simulink model "slosh_control_loop"  (R2025b)
settings: Solver=ode45  StartTime=0.0  StopTime=20  RelTol=1e-3
values from neighbouring files (symbols this model uses):
  A_mimo = A    [LQR_Tuning.m]
  A_slosh = [0, 1; -k_slosh/m_slosh_comp, -b_slosh/m_slosh_comp]    [adaptive_pid_vs_lqi_comparison.m]    (also in comprehensive_slosh_analysis.m = [0, 1; -k_slosh_comp/m_slosh_comp, -b_slosh_comp/m_slosh_com; improved_physics_slosh_model.m; separated_architecture.m = [0,                1; separated_system_params.mat = [0  1; -4  -0.2])
  B_nom = [B_mimo,B_nom(:,3),B_nom(:,4)]    [LQR_Tuning.m]    (also in adaptive_pid_vs_lqi_comparison.m = [0,     0; comprehensive_slosh_analysis.m = [0,     0; improved_physics_slosh_model.m = [0,     0; separated_architecture.m = [1/m_aircraft,  XT/m_aircraft, 1/m_aircraft,      0)
  B_slosh = [0; 1]    [adaptive_pid_vs_lqi_comparison.m]    (also in comprehensive_slosh_analysis.m; improved_physics_slosh_model.m; separated_architecture.m = [0,           0; separated_system_params.mat = [0  0; 1  1.5])
  C_nom = eye(4)    [separated_architecture.m]    (also in separated_system_params.mat = [1 0 0 0 0 1 0 0 0 0 1 0 ... (16 elements, 4x4)])
  C_slosh = eye(2)    [separated_architecture.m]    (also in separated_system_params.mat = [1  0; 0  1])
  D_nom = zeros(4, 4)    [separated_architecture.m]    (also in separated_system_params.mat = [0 0 0 0 0 0 0 0 0 0 0 0 ... (16 elements, 4x4)])
  K_aug = lqr(A_aug, B_aug, Q_aug, R_aug)    [LQR_Tuning.m]    (also in adaptive_pid_vs_lqi_comparison.m; comprehensive_slosh_analysis.m; improved_physics_slosh_model.m; lqi_controller.mat = [2.96092993839  3.51939058392  1.16330734003  0.040446521077)
settings Model: Creator=piepe  LastModifiedBy=pieper

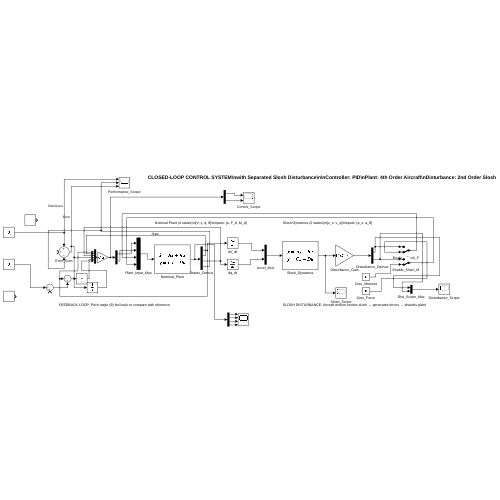
[thumbnail: Simulink's stored preview of the top-level diagram]
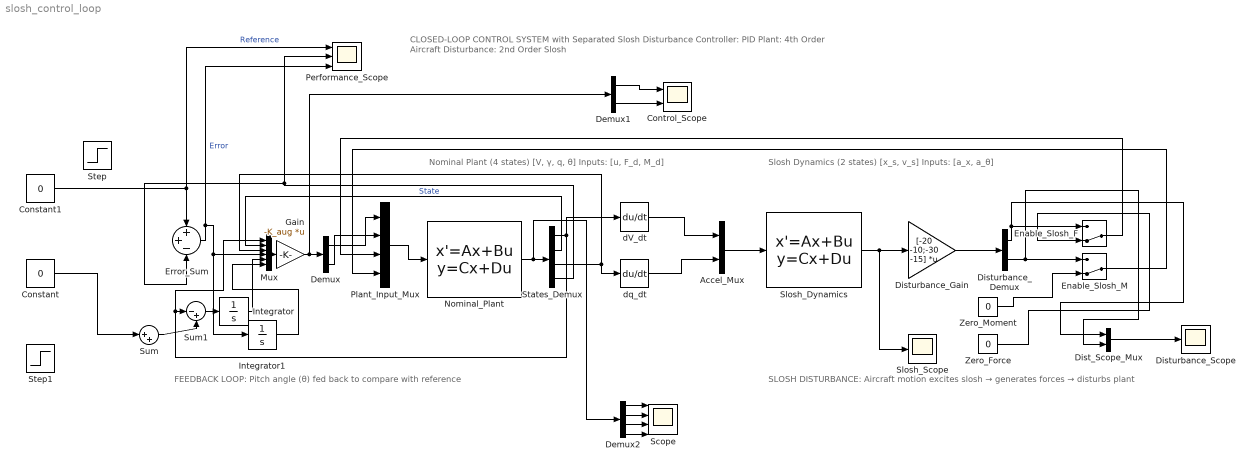
== system slosh_control_loop ==
  note: Nominal Plant (4 states)\n[V, γ, q, θ]\nInputs: [u, F_d, M_d]
  note: Slosh Dynamics (2 states)\n[x_s, v_s]\nInputs: [a_x, a_θ]
  note: CLOSED-LOOP CONTROL SYSTEM\nwith Separated Slosh Disturbance\n\nController: PID\nPlant: 4th Order Aircraft\nDisturbance: 2nd Order Slosh
  note: FEEDBACK LOOP: Pitch angle (θ) fed back to compare with reference
  note: SLOSH DISTURBANCE: Aircraft motion excites slosh → generates forces → disturbs plant
  Accel_Mux : Mux  Inputs=2
  Constant : Constant  Value=0
  Constant1 : Constant  Value=0
  Control_Scope : Scope  NumInputPorts=2
      settings: ActiveDisplayYMinimum=-1  ActiveDisplayYMaximum=1
  Demux : Demux  Outputs=2
  Demux1 : Demux  Outputs=2
  Demux2 : Demux
  Dist_Scope_Mux : Mux  Inputs=2
  Disturbance_Demux : Demux  Outputs=2
  Disturbance_Gain : Gain  Gain=[-20 -10;-30 -15]  Multiplication=Matrix(K*u)
  Disturbance_Scope : Scope
      settings: ActiveDisplayYMinimum=-1  ActiveDisplayYMaximum=1
  Enable_Slosh_F : ManualSwitch  CurrentSetting=0
  Enable_Slosh_M : ManualSwitch  CurrentSetting=0
  Error_Sum : Sum  Inputs=++-
  Gain : Gain  Gain=-K_aug  Multiplication=Matrix(K*u)
  Integrator : Integrator
  Integrator1 : Integrator
  Mux : Mux  Inputs=6
  Nominal_Plant : StateSpace  A=A_mimo  B=B_nom  C=C_nom  D=D_nom  InitialCondition=[0;0;0;0]
  Performance_Scope : Scope  NumInputPorts=3
      settings: ActiveDisplayYMinimum=-1  ActiveDisplayYMaximum=1
  Plant_Input_Mux : Mux
  Scope : Scope  NumInputPorts=4
      settings: ActiveDisplayYMinimum=-1  ActiveDisplayYMaximum=1
  Slosh_Dynamics : StateSpace  A=A_slosh  B=B_slosh  C=C_slosh  D=[0 0;0 0]  InitialCondition=[0.1;0]
  Slosh_Scope : Scope
  States_Demux : Demux
  Step : Step  After=0.1  SampleTime=0
  Step1 : Step  SampleTime=0
  Sum : Sum  Inputs=|++
  Sum1 : Sum  Inputs=|-+
  Zero_Force : Constant  Value=0
  Zero_Moment : Constant  Value=0
  dV_dt : Derivative
  dq_dt : Derivative
  wires:
  Constant1/1 -> Error_Sum/1, Performance_Scope/1  "Reference"
  Error_Sum/1 -> Mux/4, Integrator1/1, Performance_Scope/3  "Error"
  Plant_Input_Mux/1 -> Nominal_Plant/1
  Nominal_Plant/1 -> Demux2/1, States_Demux/1
  States_Demux/4 -> Error_Sum/3, Performance_Scope/2  "State"
  States_Demux/3 -> Mux/3, dq_dt/1
  dV_dt/1 -> Accel_Mux/1
  dq_dt/1 -> Accel_Mux/2
  Accel_Mux/1 -> Slosh_Dynamics/1
  Slosh_Dynamics/1 -> Disturbance_Gain/1, Slosh_Scope/1
  Disturbance_Gain/1 -> Disturbance_Demux/1
  Disturbance_Demux/1 -> Enable_Slosh_F/1, Dist_Scope_Mux/1
  Disturbance_Demux/2 -> Enable_Slosh_M/1, Dist_Scope_Mux/2
  Zero_Force/1 -> Enable_Slosh_F/2
  Zero_Moment/1 -> Enable_Slosh_M/2
  Enable_Slosh_F/1 -> Plant_Input_Mux/3
  Enable_Slosh_M/1 -> Plant_Input_Mux/4
  Dist_Scope_Mux/1 -> Disturbance_Scope/1
  Mux/1 -> Gain/1
  Gain/1 -> Demux1/1, Demux/1
  Demux/1 -> Plant_Input_Mux/1
  Demux/2 -> Plant_Input_Mux/2
  States_Demux/1 -> dV_dt/1, Mux/1, Sum1/1
  States_Demux/2 -> Mux/2
  Demux1/1 -> Control_Scope/1
  Demux1/2 -> Control_Scope/2
  Demux2/1 -> Scope/1
  Demux2/2 -> Scope/2
  Demux2/3 -> Scope/3
  Demux2/4 -> Scope/4
  Sum1/1 -> Integrator/1
  Integrator/1 -> Mux/5
  Integrator1/1 -> Mux/6
  Sum/1 -> Sum1/2
  Constant/1 -> Sum/1
